simulink model "Batman_Code"  (Simulink 7.8)
settings: Solver=FixedStepDiscrete  StartTime=0.0  StopTime=3  FixedStep=0.000250  RelTol=1e-3
InitFcn:
  | if (rtwenvironmentmode(bdroot(gcbh)) || ...
  |       exist('sldvisactive','file')~=0 && ...
  |       sldvisactive(bdroot(gcbh)) )
  |    ; %Simulation
  | else
  |   SendTargetStop(); %RTW-Build
  | end
values from neighbouring files (symbols this model uses):
  A = diag([ 1  (1-T_s/(C_dl*R_dl))])    [Batman_Code_param.m]
  A_T = A'    [Batman_Code_param.m]
  B = [(T_s/C_cell);  (T_s/C_dl) ]    [Batman_Code_param.m]
  CellNo = uint8(12)    [Batman_Code_param.m]    (also in Init_file_Bat.m = uint16(12))
  I_max_line = int32(100000)    [Batman_Code_param.m]    (also in Init_file_Bat.m = int32(10000))
  I_min_line = int32(-100000)    [Batman_Code_param.m]    (also in Init_file_Bat.m = int32(-10000))
  max_delta_V_cell = uint16(100)    [Batman_Code_param.m]
  p = [2.2966e-006 -3.6644e-004 0.0252 2.9036]'    [Batman_Code_param.m]
  P_0 = [1e-5 8e-8; 8e-8 1.4e-8]    [Batman_Code_param.m]
  Q = diag( B.^2 .* stddev_I_k^2 )    [Batman_Code_param.m]
  R = stddev_V_k^2    (= 1.00195407867e-06)    [Batman_Code_param.m]
  R_i = 0.05    [Batman_Code_param.m]    (also in Init_file_Bat.m = 0.002)
  T_max_cell = uint16(373)    [Batman_Code_param.m]    (also in Init_file_Bat.m)
  T_min_cell = uint16(273)    [Batman_Code_param.m]    (also in Init_file_Bat.m)
  V_max_bat = uint16(49200)    [Batman_Code_param.m]    (also in Init_file_Bat.m = uint16(49080))
  V_max_cell = uint16(4090)    [Batman_Code_param.m]    (also in Init_file_Bat.m)
  V_min_bat = uint16(30000)    [Batman_Code_param.m]    (also in Init_file_Bat.m = uint16(36000))
  V_min_cell = uint16(3000)    [Batman_Code_param.m]    (also in Init_file_Bat.m = uint16(2800))
undefined symbols (not defined in the file or in its folder): BlockLoadFcnInfoBlock
libraries: c280xlib x20, lucasnuelle x2, idelinklib_ticcs x1, c2833xlib x1, idelinklib_tgtpref x1, idelinklib_common x1
(part 1 of 2)
settings Model: Creator=mathlab  LastModifiedBy=user  BufferReuse=off
settings SolverCC: AutoInsertRateTranBlk=on
settings DataIOCC: SaveOutput=off  SaveTime=off
settings OptimizationCC: BlockReduction=off  InlineParams=on  BufferReuse=off  OptimizeModelRefInitCode=on  LifeSpan=1
settings DebuggingCC: MultiTaskDSMMsg=none  MultiTaskCondExecSysMsg=none  UniqueDataStoreMsg=warning  SFNoUnconditionalDefaultTransitionDiag=none
settings HardwareCC: ProdBitPerChar=16  ProdBitPerInt=16  ProdBitPerPointer=16  ProdLargestAtomicInteger=Integer  ProdIntDivRoundTo=Zero  ProdEndianess=LittleEndian  ProdWordSize=16  ProdHWDeviceType=Texas Instruments->C2000
settings RTWCC: SystemTargetFile=idelink_ert.tlc  TLCOptions=-v  GenerateMakefile=off  TemplateMakefile=idelink_ert.tmf  PostCodeGenCommand=LNPostCodeGenCommand(modelName, buildInfo)  Description=IDE Link ERT  ProcessScript=idelink_ert_make_rtw_hook
settings CodeAppCC: IgnoreCustomStorageClasses=off
settings ERTFactory: TargetFcnLib=ansi_tfl_table_tmw.mat  TargetFunctionLibrary=ANSI_C  UtilityFuncGeneration=Auto  ERTMultiwordTypeDef=System defined  CodeExecutionProfiling=off  ERTMultiwordLength=256  MultiwordLength=2048  GenerateFullHeader=on  GenerateSampleERTMain=off  GenerateTestInterfaces=off  IsPILTarget=off  ModelReferenceCompliant=on  ParMdlRefBuildCompliant=off  CompOptLevelCompliant=off  ConcurrentExecutionCompliant=on  IncludeMdlTerminateFcn=on  GeneratePreprocessorConditionals=Disable all  CombineOutputUpdateFcns=on  CombineSignalStateStructs=off  SuppressErrorStatus=off  ERTFirstTimeCompliant=on  IncludeFileDelimiter=Auto  ERTCustomFileBanners=on  SupportAbsoluteTime=on  LogVarNameModifier=rt_  MatFileLogging=off  MultiInstanceERTCode=off  SupportNonFinite=on  SupportComplex=on  PurelyIntegerCode=off  SupportContinuousTime=off  SupportNonInlinedSFcns=on  SupportVariableSizeSignals=off  EnableShiftOperators=on  ParenthesesLevel=Nominal  PortableWordSizes=off  ModelStepFunctionPrototypeControlCompliant=on  CPPClassGenCompliant=off  AutosarCompliant=off  GenerateErtSFunction=off  CreateSILPILBlock=None  CodeExecutionProfileVariable=executionProfile  CodeProfilingSaveOptions=SummaryOnly  GenerateASAP2=off  ExtMode=off  ExtModeTransport=0  ExtModeStaticAlloc=off  ExtModeStaticAllocSize=1000000  ExtModeTesting=off  ExtModeMexFile=TIC2000ExternalModeOpen  ExtModeIntrfLevel=Level2 - Open  InlinedParameterPlacement=Hierarchical  TargetOS=BareBoardExample  MultiInstanceErrorCode=Error  RateGroupingCode=on  RootIOFormat=Individual arguments  RTWCAPISignals=off  RTWCAPIParams=off  RTWCAPIStates=off  RTWCAPIRootIO=off  ERTSrcFileBannerTemplate=ert_code_template.cgt  ERTHdrFileBannerTemplate=ert_code_template.cgt  ERTDataSrcFileTemplate=ert_code_template.cgt  ERTDataHdrFileTemplate=ert_code_template.cgt  ERTCustomFileTemplate=example_file_process.tlc  CoverageDialogOpen=off  EnableDataOwnership=off  SignalDisplayLevel=10  ParamTuneLevel=10  GlobalDataDefinition=Auto  DataDefinitionFile=global.c  GlobalDataReference=Auto  ERTFilePackagingFormat=Modular  DataReferenceFile=global.h  GRTInterface=off  PreserveExpressionOrder=off  PreserveIfCondition=off  ConvertIfToSwitch=off  PreserveExternInFcnDecls=on  SuppressUnreachableDefaultCases=off  EnableUserReplacementTypes=off  MemSecPackage=--- None ---  MemSecDataConstants=Default  MemSecDataIO=Default  MemSecDataInternal=Default  MemSecDataParameters=Default  MemSecFuncInitTerm=Default  MemSecFuncExecute=Default  MemSecFuncSharedUtil=Default  CodeProfilingInstrumentation=off  AdaptorName=Texas Instruments Code Composer Studio v4 (makefile generation only)  exportIDEObj=on  ideObjName=IDE_Obj  oldideObjName=IDE_Obj  ideObjTimeout=1000  oldideObjTimeout=1000  ideObjBuildTimeout=1000  oldideObjBuildTimeout=1000  ProfileGenCode=off  profileBy=Tasks  ProfileNumSamples=100  InlineDSPBlks=off  projectOptions=Release  debugCompilerOptions=-s -O2 -dDSP=1  releaseCompilerOptions=-s -O2 -dDSP=1  compilerOptionsStr=-s -O2 -dDSP=1  getCompilerOptions=off  resetCompilerOptions=off  debugLinkerOptions=-heap0x10000 -ecode_start -q  releaseLinkerOptions=-heap0x10000 -ecode_start -q  linkerOptionsStr=-heap0x10000 -ecode_start -q  getLinkerOptions=off  resetLinkerOptions=off  systemStackSize=600  systemHeapSize=512  buildFormat=Makefile  buildAction=Create  overrunNotificationMethod=None  overrunNotificationFcn=myfunction  oldoverrunNotificationFcn=myfunction  configurePIL=off  configPILBlockAction=None  DiagnosticActions=warning

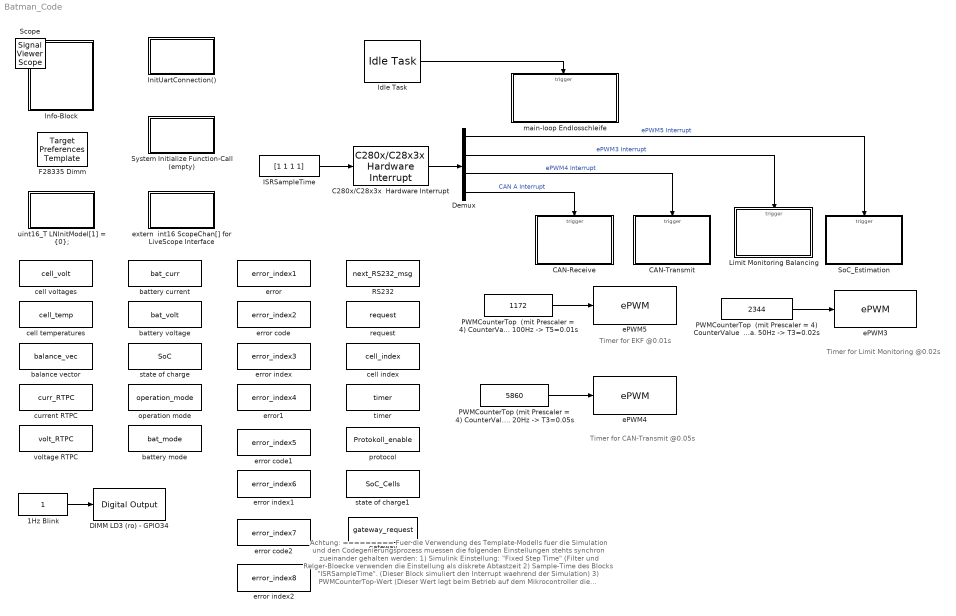
== system Batman_Code ==
  note: Achtung:
      | =========
      | Fuer die Verwendung des Template-Modells fuer die Simulation und den Codegenierungsprozess
      | muessen die folgenden Einstellungen stehts synchron zueinander gehalten werden:
      |
      | 1) Simulink Einstellung: "Fixed Step Time"          (Filter und Relger-Bloecke verwenden die Einstellung als diskrete Abtastzeit
      | 2) Sample-Time des Blocks "ISRSampleTime".   (Dieser Block simuliert den Interrupt waehrend der Simulation)
      | 3) PWMCounterTop-Wert                                    (Dieser Wert legt beim Betrieb auf dem Mikrocontroller die Interrupt-Aufrufzeit fest)
      |                                                                            --> Wert = 150Mhz/(4 * FREQUENZ)
      | Beispiel 4kHz:
      | -------------------------
      | Simulink-Einstellung "FixedStep Time":  0.000250
      | Sample-Time ISRSampleTime-Block:     0.000250
      | PWMCounterTop:                                 150Mhz/(4*4kHz) = 9375
      |
      | Achtung:
      | ==========
      | Werden mehrere Interrupt-Service-Routinen verwendet (hinzugefuegt) muss in jede ISR (Subsystem) der Block: "System Output",
      | wie dieser in den bereits vorhandenen ISRs vorkommt kopiert werden, damit die Oszilloskopfunktion die hoechste Prioritaet besitzt!
  note: Timer for EKF @0.01s
  note: Timer for Limit
      | Monitoring @0.02s
  note: Timer for
      | CAN-Transmit @0.05s
  1Hz Blink : Constant  SampleTime=1
  C280x/C28x3x  Hardware Interrupt : idelinklib_ticcs/C280x//C28x3x Hardware Interrupt  irqnumbers=[3 3 3 9]  pienumbers=[5 3 4 6]  irqpriorities=[99 97 90 80]  irqpreempts=[0 1 0 1]  showinput=on  dspchiptype=C280X
  CAN-Receive : Subsystem  TreatAsAtomicUnit=on
  CAN-Transmit : Subsystem  TreatAsAtomicUnit=on
  DIMM LD3 (ro) - GPIO34 : c2833xlib/Digital Output  GPIO_Number=GPIO32~GPIO39  GPIO_Bit0=off  GPIO_BIT0_Toggle=off  GPIO_Bit1=off  GPIO_BIT1_Toggle=off  GPIO_Bit2=on  GPIO_BIT2_Toggle=on  GPIO_Bit3=off  GPIO_BIT3_Toggle=off  GPIO_Bit4=off  GPIO_BIT4_Toggle=off  GPIO_Bit5=off  GPIO_BIT5_Toggle=off  GPIO_Bit6=off  GPIO_BIT6_Toggle=off  GPIO_Bit7=off  GPIO_BIT7_Toggle=off
  Demux : Demux
  F28335 Dimm : idelinklib_tgtpref/Target Preferences Template  Tag=ccslinktgtpref_ccsv4  library=off
  ISRSampleTime : Constant  Value=[1 1 1 1]  SampleTime=0.000250
  Idle Task : idelinklib_common/Idle Task  tasknumbers=[1]  taskpriorities=100017  taskpreempts=[1]  showinput=off  simPriority=0
  Info-Block : Subsystem  LoadFcn=BlockLoadFcnInfoBlock(gcb);  TreatAsAtomicUnit=on  mask{version=unused, date=unused, modelDescription=unused, hardware=unused, comInterface=LNComFTDI2232, displaySupport=unused, ccssupport=Code Composer Studio 5 (Lucas-Nülle Support), ccstargetconfiguration=C2000 F28335 XDS100V1, ccsmemorymap=F28335 bulk ram}
      mask prompts: version "Modell-Version:"; date "Build-Date:"; modelDescription "Description:"; hardware "Usage for Hardware:"; comInterface "Communication-Interface:"; displaySupport "Display Support:"; ccssupport "Code Composer Studio Support:"; ccstargetconfiguration "Target Configuration:"; ccsmemorymap "Used Memory Map Configuration:"
      mask init:
      | set_param(gcb, 'MaskSelfModifiable', 'on');
      mask StyleString: edit,edit,edit,edit,edit,edit,popup(Code Composer Studio 3.3|Code Composer Studio 5 (Lucas-Nülle Support)),popup(C2000 F28335 XDS100V2|C2000 F28335 XDS100V1|C2000 F28335 XDS100V3|C2000 F28335 XDS200USB|C2000 F28335 XDS510LC|C2000 F28335 XDS510USB|C2000 F28335 XDS560V2USB),popup(System Settings|F28335 External SRAM 512kB|F28335 bulk flash|F28335 bulk ram)
  InitUartConnection() : Subsystem  mask(System Initialize){ShowInLibBrowser=0}
      mask prompts: ShowInLibBrowser "Mask Parameter 1:"
      mask help: Add code to a systems Initialize function
      settings: CopyFcn=cccopyfcn(gcb)  OpenFcn=ccopenfcn('System Initialize Function')
      mask Help: eval('feval(''rtwprivate'',''rtwhelpview'',''rtw_sys_initialize_block'')');
      mask Display: disp('System\nInitialize');
  Limit Monitoring Balancing : Subsystem  TreatAsAtomicUnit=on
  "PWMCounterTop  (mit Prescaler = 4) CounterValue  = 150MHz / (128*10*Freqeuenz) 1172 -> ca. 100Hz -> T5=0.01s" : Constant  Value=1172  OutDataTypeStr=uint32
  "PWMCounterTop  (mit Prescaler = 4) CounterValue  = 150MHz / (128*10*Freqeuenz) 2344 -> ca. 50Hz -> T3=0.02s" : Constant  Value=2344  OutDataTypeStr=uint32
  "PWMCounterTop (mit Prescaler = 4) CounterValue  = 150MHz / (128*10*Freqeuenz) 5860 -> ca. 20Hz -> T3=0.05s" : Constant  Value=5860  OutDataTypeStr=uint32
  RS232 : DataStoreMemory  DataStoreName=next_RS232_msg  ReadBeforeWriteMsg=warning  WriteAfterWriteMsg=warning  WriteAfterReadMsg=warning  InitialValue=1  OutDataTypeStr=boolean
  SoC_Estimation : Subsystem  TreatAsAtomicUnit=on
  System Initialize Function-Call (empty) : Subsystem  mask(System Initialize){ShowInLibBrowser=0}
      mask prompts: ShowInLibBrowser "Mask Parameter 1:"
      mask help: Add code to a systems Initialize function
      settings: CopyFcn=cccopyfcn(gcb)  OpenFcn=ccopenfcn('System Initialize Function')
      mask Help: eval('feval(''rtwprivate'',''rtwhelpview'',''rtw_sys_initialize_block'')');
      mask Display: disp('System\nInitialize');
  balance vector : DataStoreMemory  DataStoreName=balance_vec  ReadBeforeWriteMsg=warning  WriteAfterWriteMsg=warning  WriteAfterReadMsg=warning  InitialValue=zeros(CellNo,1)  OutDataTypeStr=uint8
  battery current : DataStoreMemory  DataStoreName=bat_curr  ReadBeforeWriteMsg=warning  WriteAfterWriteMsg=warning  WriteAfterReadMsg=warning  OutDataTypeStr=int16
  battery mode : DataStoreMemory  DataStoreName=bat_mode  ReadBeforeWriteMsg=warning  WriteAfterWriteMsg=warning  WriteAfterReadMsg=warning  InitialValue=1  OutDataTypeStr=uint16
  battery voltage : DataStoreMemory  DataStoreName=bat_volt  ReadBeforeWriteMsg=warning  WriteAfterWriteMsg=warning  WriteAfterReadMsg=warning  OutDataTypeStr=uint16
  cell index : DataStoreMemory  DataStoreName=cell_index  ReadBeforeWriteMsg=warning  WriteAfterWriteMsg=warning  WriteAfterReadMsg=warning  InitialValue=[0 0]  OutDataTypeStr=uint8
  cell temperatures : DataStoreMemory  DataStoreName=cell_temp  ReadBeforeWriteMsg=warning  WriteAfterWriteMsg=warning  WriteAfterReadMsg=warning  InitialValue=zeros(CellNo,1)  OutDataTypeStr=uint16
  "cell voltages " : DataStoreMemory  DataStoreName=cell_volt  ReadBeforeWriteMsg=warning  WriteAfterWriteMsg=warning  WriteAfterReadMsg=warning  InitialValue=zeros(CellNo,1)  OutDataTypeStr=uint16
  current RTPC : DataStoreMemory  DataStoreName=curr_RTPC  ReadBeforeWriteMsg=warning  WriteAfterWriteMsg=warning  WriteAfterReadMsg=warning  InitialValue=500  OutDataTypeStr=int16
  ePWM3 : c280xlib/ePWM  checkMode=off  useModule=ePWM3  periodUnits=Clock cycles  timerSource=Input port  timerPeriod_clk=0  timerPeriod_sec=PwmTsample  countingMode=Up  synchronizationOption=Disable  synchronizationEnable=off  phaseActiveEnable=Disable  phaseDirection=Count down after sync  phaseActive=0  clockPrescale=128  HSclockPrescale=10  ePWMxAStatus=off  CMPAUnits=Percentages  CMPASource=Specify via dialog  CMPAValue_per=50  CMPAValue_clk=5000  ePWMxAactionLogic1=Clear  ePWMxAactionLogic2=Do nothing  ePWMxAactionLogic3=Set  ePWMxAactionLogic4=Do nothing  ePWMxAactionLogic5=Do nothing  ePWMxAactionLogic6=Do nothing  ePWMxALoadMode=Load on CTR=Zero  ePWMxACSFenable=off  ePWMxACSFvalue=Forcing Disable  ePWMxASFreload=Zero  enHRPWM=off  HRPWM_LoadMode=CTR=ZERO  HRPWM_CTLMode=Phase control mode  HRPWM_EDGMode=Both edge  enSFO=on  ePWMxBStatus=off  CMPBUnits=Percentages  CMPBSource=Specify via dialog  CMPBValue_per=0  CMPBValue_clk=0  ePWMxBactionLogic1=Do nothing  ePWMxBactionLogic2=Set  ePWMxBactionLogic3=Do nothing  ePWMxBactionLogic4=Do nothing  ePWMxBactionLogic5=Clear  ePWMxBactionLogic6=Do nothing  ePWMxBLoadMode=Load on CTR=Zero  ePWMxBCSFenable=off  ePWMxBCSFvalue=Forcing Disable  ePWMxBSFreload=Zero  enableDBePWMxA=off  enableDBePWMxB=off  DBpolarity=AH  DBedgeDelay=Positive  DBSource_ePWMxA=ePWMxA  DBSource_ePWMxB=ePWMxA  DBperiodSource=Specify via dialog  REDperiod=0  FEDperiod=0  adcstartModuleA=off  adcrequestEventA=First event  adcstartEventA=CTR=Zero  adcstartModuleB=off  adcrequestEventB=First event  adcstartEventB=CTR=Zero  intEn=on  intPrd=First event  intSel=CTR=PRD  chopperEnable=off  chopperFrequency=1  chopperFirstwidth=1  chopperDuty=12.5%  tripZonesource=Specify via dialog  tzselOSHT1=off  tzselOSHT2=off  tzselOSHT3=off  tzselOSHT4=off  tzselOSHT5=off  tzselOSHT6=off  tzselCBC1=off  tzselCBC2=off  tzselCBC3=off  tzselCBC4=off  tzselCBC5=off  tzselCBC6=off  enTzOstIntr=off  enTzCbcIntr=off  ePWMxAforced=No action  ePWMxBforced=No action  timerPeriod=-1  ePWMxAValue=1  ePWMxBValue=0  tripZoneoption=OSHT
  ePWM4 : c280xlib/ePWM  checkMode=off  useModule=ePWM4  periodUnits=Clock cycles  timerSource=Input port  timerPeriod_clk=0  timerPeriod_sec=PwmTsample  countingMode=Up  synchronizationOption=Disable  synchronizationEnable=off  phaseActiveEnable=Disable  phaseDirection=Count down after sync  phaseActive=0  clockPrescale=128  HSclockPrescale=10  ePWMxAStatus=off  CMPAUnits=Percentages  CMPASource=Specify via dialog  CMPAValue_per=50  CMPAValue_clk=5000  ePWMxAactionLogic1=Clear  ePWMxAactionLogic2=Do nothing  ePWMxAactionLogic3=Set  ePWMxAactionLogic4=Do nothing  ePWMxAactionLogic5=Do nothing  ePWMxAactionLogic6=Do nothing  ePWMxALoadMode=Load on CTR=Zero  ePWMxACSFenable=off  ePWMxACSFvalue=Forcing Disable  ePWMxASFreload=Zero  enHRPWM=off  HRPWM_LoadMode=CTR=ZERO  HRPWM_CTLMode=Phase control mode  HRPWM_EDGMode=Both edge  enSFO=on  ePWMxBStatus=off  CMPBUnits=Percentages  CMPBSource=Specify via dialog  CMPBValue_per=0  CMPBValue_clk=0  ePWMxBactionLogic1=Do nothing  ePWMxBactionLogic2=Set  ePWMxBactionLogic3=Do nothing  ePWMxBactionLogic4=Do nothing  ePWMxBactionLogic5=Clear  ePWMxBactionLogic6=Do nothing  ePWMxBLoadMode=Load on CTR=Zero  ePWMxBCSFenable=off  ePWMxBCSFvalue=Forcing Disable  ePWMxBSFreload=Zero  enableDBePWMxA=off  enableDBePWMxB=off  DBpolarity=AH  DBedgeDelay=Positive  DBSource_ePWMxA=ePWMxA  DBSource_ePWMxB=ePWMxA  DBperiodSource=Specify via dialog  REDperiod=0  FEDperiod=0  adcstartModuleA=off  adcrequestEventA=First event  adcstartEventA=CTR=Zero  adcstartModuleB=off  adcrequestEventB=First event  adcstartEventB=CTR=Zero  intEn=on  intPrd=First event  intSel=CTR=PRD  chopperEnable=off  chopperFrequency=1  chopperFirstwidth=1  chopperDuty=12.5%  tripZonesource=Specify via dialog  tzselOSHT1=off  tzselOSHT2=off  tzselOSHT3=off  tzselOSHT4=off  tzselOSHT5=off  tzselOSHT6=off  tzselCBC1=off  tzselCBC2=off  tzselCBC3=off  tzselCBC4=off  tzselCBC5=off  tzselCBC6=off  enTzOstIntr=off  enTzCbcIntr=off  ePWMxAforced=No action  ePWMxBforced=No action  timerPeriod=-1  ePWMxAValue=1  ePWMxBValue=0  tripZoneoption=OSHT
  ePWM5 : c280xlib/ePWM  checkMode=off  useModule=ePWM5  periodUnits=Clock cycles  timerSource=Input port  timerPeriod_clk=0  timerPeriod_sec=PwmTsample  countingMode=Up  synchronizationOption=Disable  synchronizationEnable=off  phaseActiveEnable=Disable  phaseDirection=Count down after sync  phaseActive=0  clockPrescale=128  HSclockPrescale=10  ePWMxAStatus=off  CMPAUnits=Percentages  CMPASource=Specify via dialog  CMPAValue_per=50  CMPAValue_clk=5000  ePWMxAactionLogic1=Clear  ePWMxAactionLogic2=Do nothing  ePWMxAactionLogic3=Set  ePWMxAactionLogic4=Do nothing  ePWMxAactionLogic5=Do nothing  ePWMxAactionLogic6=Do nothing  ePWMxALoadMode=Load on CTR=Zero  ePWMxACSFenable=off  ePWMxACSFvalue=Forcing Disable  ePWMxASFreload=Zero  enHRPWM=off  HRPWM_LoadMode=CTR=ZERO  HRPWM_CTLMode=Phase control mode  HRPWM_EDGMode=Both edge  enSFO=on  ePWMxBStatus=off  CMPBUnits=Percentages  CMPBSource=Specify via dialog  CMPBValue_per=0  CMPBValue_clk=0  ePWMxBactionLogic1=Do nothing  ePWMxBactionLogic2=Set  ePWMxBactionLogic3=Do nothing  ePWMxBactionLogic4=Do nothing  ePWMxBactionLogic5=Clear  ePWMxBactionLogic6=Do nothing  ePWMxBLoadMode=Load on CTR=Zero  ePWMxBCSFenable=off  ePWMxBCSFvalue=Forcing Disable  ePWMxBSFreload=Zero  enableDBePWMxA=off  enableDBePWMxB=off  DBpolarity=AH  DBedgeDelay=Positive  DBSource_ePWMxA=ePWMxA  DBSource_ePWMxB=ePWMxA  DBperiodSource=Specify via dialog  REDperiod=0  FEDperiod=0  adcstartModuleA=off  adcrequestEventA=First event  adcstartEventA=CTR=Zero  adcstartModuleB=off  adcrequestEventB=First event  adcstartEventB=CTR=Zero  intEn=on  intPrd=First event  intSel=CTR=PRD  chopperEnable=off  chopperFrequency=1  chopperFirstwidth=1  chopperDuty=12.5%  tripZonesource=Specify via dialog  tzselOSHT1=off  tzselOSHT2=off  tzselOSHT3=off  tzselOSHT4=off  tzselOSHT5=off  tzselOSHT6=off  tzselCBC1=off  tzselCBC2=off  tzselCBC3=off  tzselCBC4=off  tzselCBC5=off  tzselCBC6=off  enTzOstIntr=off  enTzCbcIntr=off  ePWMxAforced=No action  ePWMxBforced=No action  timerPeriod=-1  ePWMxAValue=1  ePWMxBValue=0  tripZoneoption=OSHT
  error : DataStoreMemory  DataStoreName=error_index1  ReadBeforeWriteMsg=warning  WriteAfterWriteMsg=warning  WriteAfterReadMsg=warning  OutDataTypeStr=uint16
  error code : DataStoreMemory  DataStoreName=error_index2  ReadBeforeWriteMsg=warning  WriteAfterWriteMsg=warning  WriteAfterReadMsg=warning  OutDataTypeStr=uint16
  error code1 : DataStoreMemory  DataStoreName=error_index5  ReadBeforeWriteMsg=warning  WriteAfterWriteMsg=warning  WriteAfterReadMsg=warning  OutDataTypeStr=uint16
  error code2 : DataStoreMemory  DataStoreName=error_index7  ReadBeforeWriteMsg=warning  WriteAfterWriteMsg=warning  WriteAfterReadMsg=warning  OutDataTypeStr=uint16
  error index : DataStoreMemory  DataStoreName=error_index3  ReadBeforeWriteMsg=warning  WriteAfterWriteMsg=warning  WriteAfterReadMsg=warning  OutDataTypeStr=uint16
  error index1 : DataStoreMemory  DataStoreName=error_index6  ReadBeforeWriteMsg=warning  WriteAfterWriteMsg=warning  WriteAfterReadMsg=warning  OutDataTypeStr=uint16
  error index2 : DataStoreMemory  DataStoreName=error_index8  ReadBeforeWriteMsg=warning  WriteAfterWriteMsg=warning  WriteAfterReadMsg=warning  OutDataTypeStr=uint16
  error1 : DataStoreMemory  DataStoreName=error_index4  ReadBeforeWriteMsg=warning  WriteAfterWriteMsg=warning  WriteAfterReadMsg=warning  OutDataTypeStr=uint16
  extern  int16 ScopeChan[] for LiveScope Interface : Subsystem  mask(Model Header){ShowInLibBrowser=0}
      mask prompts: ShowInLibBrowser "Mask Parameter 1:"
      mask help: Add code to the model .h file
      settings: CopyFcn=cccopyfcn(gcb)  OpenFcn=ccopenfcn('Model Header')
      mask Help: eval('feval(''rtwprivate'',''rtwhelpview'',''rtw_model_header_block'')');
      mask Display: disp('Model\nHeader');
  "gateway " : DataStoreMemory  DataStoreName=gateway_request  ReadBeforeWriteMsg=warning  WriteAfterWriteMsg=warning  WriteAfterReadMsg=warning  OutDataTypeStr=boolean
  main-loop Endlosschleife : Subsystem  TreatAsAtomicUnit=on
  operation mode : DataStoreMemory  DataStoreName=operation_mode  ReadBeforeWriteMsg=warning  WriteAfterWriteMsg=warning  WriteAfterReadMsg=warning  InitialValue=1  OutDataTypeStr=uint16
  protocol : DataStoreMemory  DataStoreName=Protokoll_enable  ReadBeforeWriteMsg=warning  WriteAfterWriteMsg=warning  WriteAfterReadMsg=warning  InitialValue=zeros(8,1)  OutDataTypeStr=boolean
  request : DataStoreMemory  DataStoreName=request  ReadBeforeWriteMsg=warning  WriteAfterWriteMsg=warning  WriteAfterReadMsg=warning  OutDataTypeStr=uint8
  state of charge : DataStoreMemory  DataStoreName=SoC  ReadBeforeWriteMsg=warning  WriteAfterWriteMsg=warning  WriteAfterReadMsg=warning  OutDataTypeStr=uint16
  state of charge1 : DataStoreMemory  DataStoreName=SoC_Cells  ReadBeforeWriteMsg=warning  WriteAfterWriteMsg=warning  WriteAfterReadMsg=warning  InitialValue=zeros(CellNo,1)  OutDataTypeStr=uint16
  timer : DataStoreMemory  DataStoreName=timer  ReadBeforeWriteMsg=warning  WriteAfterWriteMsg=warning  WriteAfterReadMsg=warning  OutDataTypeStr=uint32
  "uint16_T LNInitModel[1] = {0};" : Subsystem  mask(Model Source){ShowInLibBrowser=0}
      mask prompts: ShowInLibBrowser "Mask Parameter 1:"
      mask help: Add code to the model .c file
      settings: CopyFcn=cccopyfcn(gcb)  OpenFcn=ccopenfcn('Model Source')
      mask Help: eval('feval(''rtwprivate'',''rtwhelpview'',''rtw_model_source_block'')');
      mask Display: disp('Model\nSource');
  voltage RTPC : DataStoreMemory  DataStoreName=volt_RTPC  ReadBeforeWriteMsg=warning  WriteAfterWriteMsg=warning  WriteAfterReadMsg=warning  InitialValue=38000  OutDataTypeStr=uint16
  Scope : SignalViewerScope  IOType=viewer  RefreshTime=0.035000
  wires:
  Idle Task/1 -> main-loop Endlosschleife/Trigger
  "PWMCounterTop  (mit Prescaler = 4) CounterValue  = 150MHz / (128*10*Freqeuenz) 1172 -> ca. 100Hz -> T5=0.01s"/1 -> ePWM5/1
  ISRSampleTime/1 -> C280x/C28x3x  Hardware Interrupt/1
  1Hz Blink/1 -> DIMM LD3 (ro) - GPIO34/1
  "PWMCounterTop  (mit Prescaler = 4) CounterValue  = 150MHz / (128*10*Freqeuenz) 2344 -> ca. 50Hz -> T3=0.02s"/1 -> ePWM3/1
  "PWMCounterTop (mit Prescaler = 4) CounterValue  = 150MHz / (128*10*Freqeuenz) 5860 -> ca. 20Hz -> T3=0.05s"/1 -> ePWM4/1
  C280x/C28x3x  Hardware Interrupt/1 -> Demux/1
  Demux/1 -> SoC_Estimation/Trigger  "ePWM5 Interrupt"
  Demux/2 -> Limit Monitoring Balancing/Trigger  "ePWM3 Interrupt"
  Demux/3 -> CAN-Transmit/Trigger  "ePWM4 Interrupt"
  Demux/4 -> CAN-Receive/Trigger  "CAN A Interrupt"

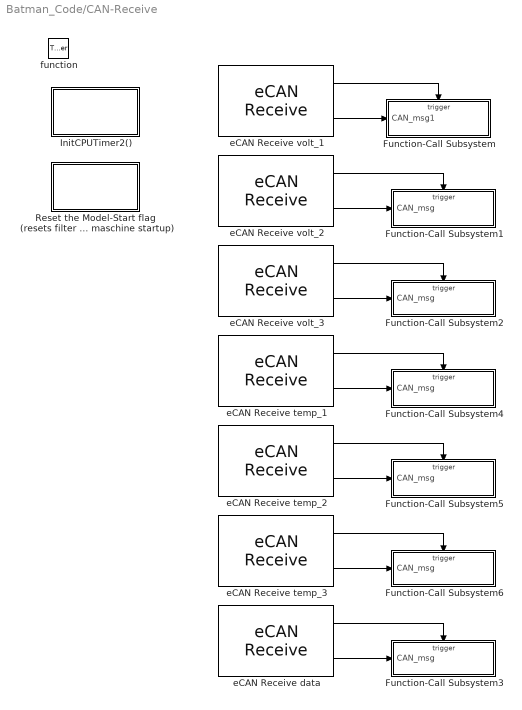
== system Batman_Code/CAN-Receive ==
  function : TriggerPort  TriggerType=function-call  SampleTime=-1
  Function-Call Subsystem : Subsystem  TreatAsAtomicUnit=on
  Function-Call Subsystem1 : Subsystem  TreatAsAtomicUnit=on
  Function-Call Subsystem2 : Subsystem  TreatAsAtomicUnit=on
  Function-Call Subsystem3 : Subsystem  TreatAsAtomicUnit=on
  Function-Call Subsystem4 : Subsystem  TreatAsAtomicUnit=on
  Function-Call Subsystem5 : Subsystem  TreatAsAtomicUnit=on
  Function-Call Subsystem6 : Subsystem  TreatAsAtomicUnit=on
  InitCPUTimer2() : Subsystem  mask(System Outputs){ShowInLibBrowser=0}
      mask prompts: ShowInLibBrowser "Mask Parameter 1:"
      mask help: Add code to a systems Outputs function
      settings: CopyFcn=cccopyfcn(gcb)  OpenFcn=ccopenfcn('System Outputs Function')
      mask Help: eval('feval(''rtwprivate'',''rtwhelpview'',''rtw_sys_outputs_block'')');
      mask Display: disp('System\nOutputs');
  Reset the Model-Start flag  (resets filter and  internal states on state  maschine startup) : Subsystem  mask(System Update){ShowInLibBrowser=0}
      mask prompts: ShowInLibBrowser "Mask Parameter 1:"
      mask help: Add code to a systems Update function
      settings: CopyFcn=cccopyfcn(gcb)  OpenFcn=ccopenfcn('System Update Function')
      mask Help: eval('feval(''rtwprivate'',''rtwhelpview'',''rtw_sys_update_block'')');
      mask Display: disp('System\nUpdate');
  eCAN Receive data : c280xlib/eCAN Receive  chipFamily=C28x3x  useModule=eCAN_A  mailboxNo=7  messageID=id_data_receive_data  messageType=Standard (11-bit identifier)  sampleTime=-1  dataType=uint32  initValue=0  outputMessageLength=off  outputMessageTimeStamp=off  postInterrupt=on  interruptLine=1
  eCAN Receive temp_1 : c280xlib/eCAN Receive  chipFamily=C28x3x  useModule=eCAN_A  mailboxNo=4  messageID=id_data_receive_temperature_1  messageType=Standard (11-bit identifier)  sampleTime=-1  dataType=uint32  initValue=0  outputMessageLength=off  outputMessageTimeStamp=off  postInterrupt=on  interruptLine=1
  eCAN Receive temp_2 : c280xlib/eCAN Receive  chipFamily=C28x3x  useModule=eCAN_A  mailboxNo=5  messageID=id_data_receive_temperature_2  messageType=Standard (11-bit identifier)  sampleTime=-1  dataType=uint32  initValue=0  outputMessageLength=off  outputMessageTimeStamp=off  postInterrupt=on  interruptLine=1
  eCAN Receive temp_3 : c280xlib/eCAN Receive  chipFamily=C28x3x  useModule=eCAN_A  mailboxNo=6  messageID=id_data_receive_temperature_3  messageType=Standard (11-bit identifier)  sampleTime=-1  dataType=uint32  initValue=0  outputMessageLength=off  outputMessageTimeStamp=off  postInterrupt=on  interruptLine=1
  eCAN Receive volt_1 : c280xlib/eCAN Receive  chipFamily=C28x3x  useModule=eCAN_A  mailboxNo=1  messageID=id_data_receive_voltage_1  messageType=Standard (11-bit identifier)  sampleTime=-1  dataType=uint32  initValue=0  outputMessageLength=off  outputMessageTimeStamp=off  postInterrupt=on  interruptLine=1
  eCAN Receive volt_2 : c280xlib/eCAN Receive  chipFamily=C28x3x  useModule=eCAN_A  mailboxNo=2  messageID=id_data_receive_voltage_2  messageType=Standard (11-bit identifier)  sampleTime=-1  dataType=uint32  initValue=0  outputMessageLength=off  outputMessageTimeStamp=off  postInterrupt=on  interruptLine=1
  eCAN Receive volt_3 : c280xlib/eCAN Receive  chipFamily=C28x3x  useModule=eCAN_A  mailboxNo=3  messageID=id_data_receive_voltage_3  messageType=Standard (11-bit identifier)  sampleTime=-1  dataType=uint32  initValue=0  outputMessageLength=off  outputMessageTimeStamp=off  postInterrupt=on  interruptLine=1
  wires:
  eCAN Receive volt_1/1 -> Function-Call Subsystem/Trigger
  eCAN Receive volt_1/2 -> Function-Call Subsystem/1(CAN_msg1)
  eCAN Receive volt_2/1 -> Function-Call Subsystem1/Trigger
  eCAN Receive volt_2/2 -> Function-Call Subsystem1/1(CAN_msg)
  eCAN Receive volt_3/1 -> Function-Call Subsystem2/Trigger
  eCAN Receive volt_3/2 -> Function-Call Subsystem2/1(CAN_msg)
  eCAN Receive data/1 -> Function-Call Subsystem3/Trigger
  eCAN Receive data/2 -> Function-Call Subsystem3/1(CAN_msg)
  eCAN Receive temp_1/1 -> Function-Call Subsystem4/Trigger
  eCAN Receive temp_1/2 -> Function-Call Subsystem4/1(CAN_msg)
  eCAN Receive temp_2/1 -> Function-Call Subsystem5/Trigger
  eCAN Receive temp_2/2 -> Function-Call Subsystem5/1(CAN_msg)
  eCAN Receive temp_3/1 -> Function-Call Subsystem6/Trigger
  eCAN Receive temp_3/2 -> Function-Call Subsystem6/1(CAN_msg)

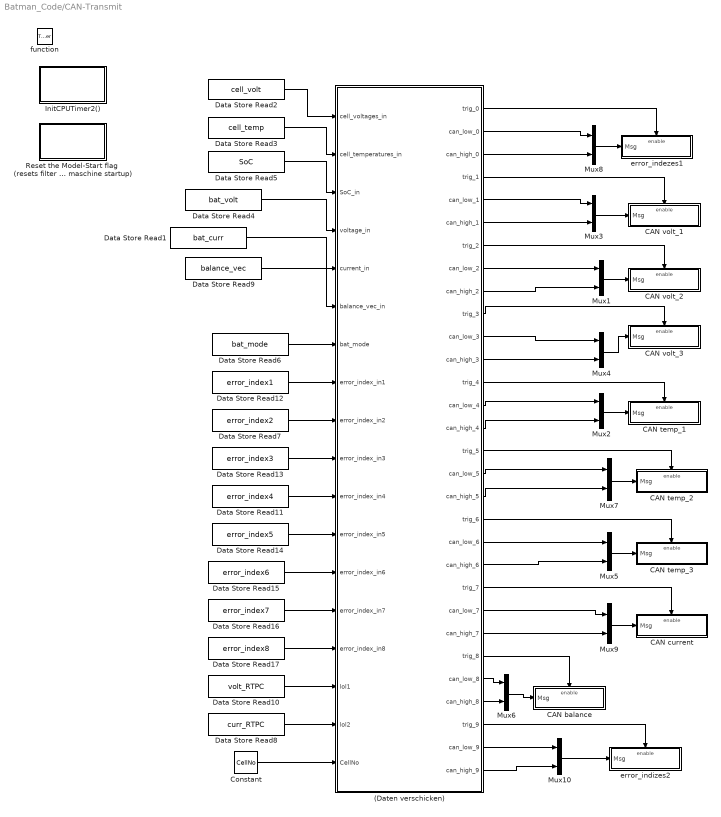
== system Batman_Code/CAN-Transmit ==
  function : TriggerPort  TriggerType=function-call  SampleTime=-1
  (Daten verschicken) : MATLAB Function  TreatAsAtomicUnit=on
  CAN balance : Subsystem  TreatAsAtomicUnit=on
  CAN current : Subsystem  TreatAsAtomicUnit=on
  CAN temp_1 : Subsystem  TreatAsAtomicUnit=on
  CAN temp_2 : Subsystem  TreatAsAtomicUnit=on
  CAN temp_3 : Subsystem  TreatAsAtomicUnit=on
  CAN volt_1 : Subsystem  TreatAsAtomicUnit=on
  CAN volt_2 : Subsystem  TreatAsAtomicUnit=on
  CAN volt_3 : Subsystem  TreatAsAtomicUnit=on
  Constant : Constant  Value=CellNo
  Data Store Read1 : DataStoreRead  DataStoreName=bat_curr
  Data Store Read10 : DataStoreRead  DataStoreName=volt_RTPC
  Data Store Read11 : DataStoreRead  DataStoreName=error_index4
  Data Store Read12 : DataStoreRead  DataStoreName=error_index1
  Data Store Read13 : DataStoreRead  DataStoreName=error_index3
  Data Store Read14 : DataStoreRead  DataStoreName=error_index5
  Data Store Read15 : DataStoreRead  DataStoreName=error_index6
  Data Store Read16 : DataStoreRead  DataStoreName=error_index7
  Data Store Read17 : DataStoreRead  DataStoreName=error_index8
  Data Store Read2 : DataStoreRead  DataStoreName=cell_volt
  Data Store Read3 : DataStoreRead  DataStoreName=cell_temp
  Data Store Read4 : DataStoreRead  DataStoreName=bat_volt
  Data Store Read5 : DataStoreRead  DataStoreName=SoC
  Data Store Read6 : DataStoreRead  DataStoreName=bat_mode
  Data Store Read7 : DataStoreRead  DataStoreName=error_index2
  Data Store Read8 : DataStoreRead  DataStoreName=curr_RTPC
  Data Store Read9 : DataStoreRead  DataStoreName=balance_vec
  InitCPUTimer2() : Subsystem  mask(System Outputs){ShowInLibBrowser=0}
      mask prompts: ShowInLibBrowser "Mask Parameter 1:"
      mask help: Add code to a systems Outputs function
      settings: CopyFcn=cccopyfcn(gcb)  OpenFcn=ccopenfcn('System Outputs Function')
      mask Help: eval('feval(''rtwprivate'',''rtwhelpview'',''rtw_sys_outputs_block'')');
      mask Display: disp('System\nOutputs');
  Mux{1..10} (10 alike) : Mux  Inputs=2
  Reset the Model-Start flag  (resets filter and  internal states on state  maschine startup) : Subsystem  mask(System Update){ShowInLibBrowser=0}
      mask prompts: ShowInLibBrowser "Mask Parameter 1:"
      mask help: Add code to a systems Update function
      settings: CopyFcn=cccopyfcn(gcb)  OpenFcn=ccopenfcn('System Update Function')
      mask Help: eval('feval(''rtwprivate'',''rtwhelpview'',''rtw_sys_update_block'')');
      mask Display: disp('System\nUpdate');
  error_indezes1 : Subsystem  TreatAsAtomicUnit=on
  error_indizes2 : Subsystem  TreatAsAtomicUnit=on
  wires:
  Mux3/1 -> CAN volt_1/1(Msg)
  Mux1/1 -> CAN volt_2/1(Msg)
  Mux4/1 -> CAN volt_3/1(Msg)
  Mux2/1 -> CAN temp_1/1(Msg)
  Mux7/1 -> CAN temp_2/1(Msg)
  Mux5/1 -> CAN temp_3/1(Msg)
  Mux9/1 -> CAN current/1(Msg)
  Mux8/1 -> error_indezes1/1(Msg)
  Mux6/1 -> CAN balance/1(Msg)
  (Daten verschicken)/2(can_low_0) -> Mux8/1
  (Daten verschicken)/3(can_high_0) -> Mux8/2
  (Daten verschicken)/1(trig_0) -> error_indezes1/Enable
  (Daten verschicken)/5(can_low_1) -> Mux3/1
  (Daten verschicken)/6(can_high_1) -> Mux3/2
  (Daten verschicken)/4(trig_1) -> CAN volt_1/Enable
  (Daten verschicken)/9(can_high_2) -> Mux1/2
  (Daten verschicken)/8(can_low_2) -> Mux1/1
  (Daten verschicken)/7(trig_2) -> CAN volt_2/Enable
  (Daten verschicken)/11(can_low_3) -> Mux4/1
  (Daten verschicken)/12(can_high_3) -> Mux4/2
  (Daten verschicken)/10(trig_3) -> CAN volt_3/Enable
  (Daten verschicken)/15(can_high_4) -> Mux2/2
  (Daten verschicken)/14(can_low_4) -> Mux2/1
  (Daten verschicken)/13(trig_4) -> CAN temp_1/Enable
  (Daten verschicken)/17(can_low_5) -> Mux7/1
  (Daten verschicken)/18(can_high_5) -> Mux7/2
  (Daten verschicken)/16(trig_5) -> CAN temp_2/Enable
  (Daten verschicken)/20(can_low_6) -> Mux5/1
  (Daten verschicken)/21(can_high_6) -> Mux5/2
  (Daten verschicken)/19(trig_6) -> CAN temp_3/Enable
  (Daten verschicken)/23(can_low_7) -> Mux9/1
  (Daten verschicken)/24(can_high_7) -> Mux9/2
  (Daten verschicken)/22(trig_7) -> CAN current/Enable
  (Daten verschicken)/26(can_low_8) -> Mux6/1
  (Daten verschicken)/27(can_high_8) -> Mux6/2
  (Daten verschicken)/25(trig_8) -> CAN balance/Enable
  Data Store Read2/1 -> (Daten verschicken)/1(cell_voltages_in)
  Data Store Read3/1 -> (Daten verschicken)/2(cell_temperatures_in)
  Data Store Read5/1 -> (Daten verschicken)/3(SoC_in)
  Data Store Read4/1 -> (Daten verschicken)/4(voltage_in)
  Data Store Read1/1 -> (Daten verschicken)/5(current_in)
  Data Store Read9/1 -> (Daten verschicken)/6(balance_vec_in)
  Data Store Read6/1 -> (Daten verschicken)/7(bat_mode)
  Data Store Read12/1 -> (Daten verschicken)/8(error_index_in1)
  Data Store Read7/1 -> (Daten verschicken)/9(error_index_in2)
  Data Store Read13/1 -> (Daten verschicken)/10(error_index_in3)
  Data Store Read10/1 -> (Daten verschicken)/16(lol1)
  Data Store Read8/1 -> (Daten verschicken)/17(lol2)
  Constant/1 -> (Daten verschicken)/18(CellNo)
  Data Store Read11/1 -> (Daten verschicken)/11(error_index_in4)
  Data Store Read14/1 -> (Daten verschicken)/12(error_index_in5)
  Data Store Read16/1 -> (Daten verschicken)/14(error_index_in7)
  Data Store Read17/1 -> (Daten verschicken)/15(error_index_in8)
  Data Store Read15/1 -> (Daten verschicken)/13(error_index_in6)
  Mux10/1 -> error_indizes2/1(Msg)
  (Daten verschicken)/29(can_low_9) -> Mux10/1
  (Daten verschicken)/30(can_high_9) -> Mux10/2
  (Daten verschicken)/28(trig_9) -> error_indizes2/Enable

== system Batman_Code/Info-Block ==

== system Batman_Code/InitUartConnection() ==

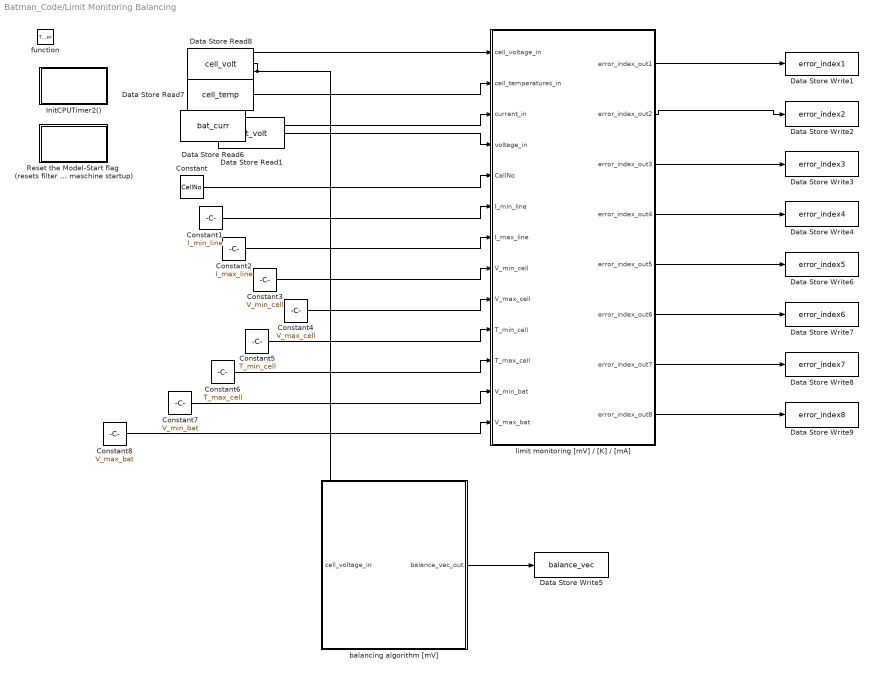
== system Batman_Code/Limit Monitoring Balancing ==
  function : TriggerPort  TriggerType=function-call  SampleTime=-1
  Constant : Constant  Value=CellNo
  Constant1 : Constant  Value=I_min_line
  Constant2 : Constant  Value=I_max_line
  Constant3 : Constant  Value=V_min_cell
  Constant4 : Constant  Value=V_max_cell
  Constant5 : Constant  Value=T_min_cell
  Constant6 : Constant  Value=T_max_cell
  Constant7 : Constant  Value=V_min_bat
  Constant8 : Constant  Value=V_max_bat
  Data Store Read1 : DataStoreRead  DataStoreName=bat_volt
  Data Store Read6 : DataStoreRead  DataStoreName=bat_curr
  Data Store Read7 : DataStoreRead  DataStoreName=cell_temp
  Data Store Read8 : DataStoreRead  DataStoreName=cell_volt
  Data Store Write1 : DataStoreWrite  DataStoreName=error_index1
  Data Store Write2 : DataStoreWrite  DataStoreName=error_index2
  Data Store Write3 : DataStoreWrite  DataStoreName=error_index3
  Data Store Write4 : DataStoreWrite  DataStoreName=error_index4
  Data Store Write5 : DataStoreWrite  DataStoreName=balance_vec
  Data Store Write6 : DataStoreWrite  DataStoreName=error_index5
  Data Store Write7 : DataStoreWrite  DataStoreName=error_index6
  Data Store Write8 : DataStoreWrite  DataStoreName=error_index7
  Data Store Write9 : DataStoreWrite  DataStoreName=error_index8
  InitCPUTimer2() : Subsystem  mask(System Outputs){ShowInLibBrowser=0}
      mask prompts: ShowInLibBrowser "Mask Parameter 1:"
      mask help: Add code to a systems Outputs function
      settings: CopyFcn=cccopyfcn(gcb)  OpenFcn=ccopenfcn('System Outputs Function')
      mask Help: eval('feval(''rtwprivate'',''rtwhelpview'',''rtw_sys_outputs_block'')');
      mask Display: disp('System\nOutputs');
  Reset the Model-Start flag  (resets filter and  internal states on state  maschine startup) : Subsystem  mask(System Update){ShowInLibBrowser=0}
      mask prompts: ShowInLibBrowser "Mask Parameter 1:"
      mask help: Add code to a systems Update function
      settings: CopyFcn=cccopyfcn(gcb)  OpenFcn=ccopenfcn('System Update Function')
      mask Help: eval('feval(''rtwprivate'',''rtwhelpview'',''rtw_sys_update_block'')');
      mask Display: disp('System\nUpdate');
  balancing algorithm [mV] : MATLAB Function  TreatAsAtomicUnit=on
  limit monitoring [mV] / [K] / [mA] : MATLAB Function  TreatAsAtomicUnit=on
  wires:
  Data Store Read6/1 -> limit monitoring [mV] / [K] / [mA]/3(current_in)
  Data Store Read8/1 -> balancing algorithm [mV]/1(cell_voltage_in), limit monitoring [mV] / [K] / [mA]/1(cell_voltage_in)
  Data Store Read7/1 -> limit monitoring [mV] / [K] / [mA]/2(cell_temperatures_in)
  limit monitoring [mV] / [K] / [mA]/1(error_index_out1) -> Data Store Write1/1
  limit monitoring [mV] / [K] / [mA]/2(error_index_out2) -> Data Store Write2/1
  balancing algorithm [mV]/1(balance_vec_out) -> Data Store Write5/1
  limit monitoring [mV] / [K] / [mA]/3(error_index_out3) -> Data Store Write3/1
  Data Store Read1/1 -> limit monitoring [mV] / [K] / [mA]/4(voltage_in)
  Constant1/1 -> limit monitoring [mV] / [K] / [mA]/6(I_min_line)
  Constant/1 -> limit monitoring [mV] / [K] / [mA]/5(CellNo)
  Constant8/1 -> limit monitoring [mV] / [K] / [mA]/13(V_max_bat)
  Constant7/1 -> limit monitoring [mV] / [K] / [mA]/12(V_min_bat)
  Constant6/1 -> limit monitoring [mV] / [K] / [mA]/11(T_max_cell)
  Constant5/1 -> limit monitoring [mV] / [K] / [mA]/10(T_min_cell)
  Constant4/1 -> limit monitoring [mV] / [K] / [mA]/9(V_max_cell)
  Constant3/1 -> limit monitoring [mV] / [K] / [mA]/8(V_min_cell)
  Constant2/1 -> limit monitoring [mV] / [K] / [mA]/7(I_max_line)
  limit monitoring [mV] / [K] / [mA]/4(error_index_out4) -> Data Store Write4/1
  limit monitoring [mV] / [K] / [mA]/5(error_index_out5) -> Data Store Write6/1
  limit monitoring [mV] / [K] / [mA]/7(error_index_out7) -> Data Store Write8/1
  limit monitoring [mV] / [K] / [mA]/8(error_index_out8) -> Data Store Write9/1
  limit monitoring [mV] / [K] / [mA]/6(error_index_out6) -> Data Store Write7/1

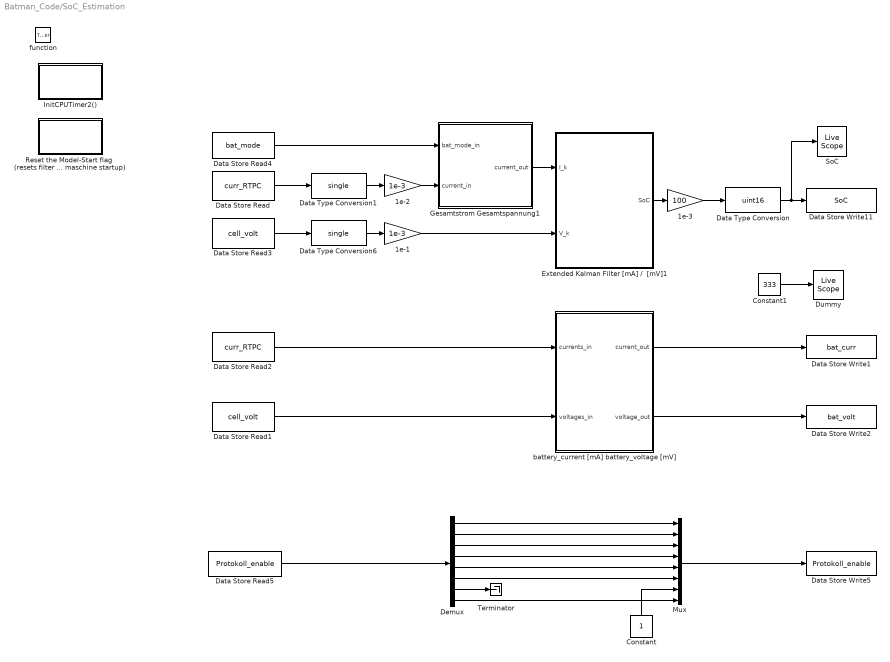
== system Batman_Code/SoC_Estimation ==
  function : TriggerPort  TriggerType=function-call  SampleTime=-1
  1e-1 : Gain  Gain=1e-3
  1e-2 : Gain  Gain=1e-3
  1e-3 : Gain  Gain=100
  Constant : Constant  OutDataTypeStr=boolean
  Constant1 : Constant  Value=333  OutDataTypeStr=uint16
  Data Store Read : DataStoreRead  DataStoreName=curr_RTPC
  Data Store Read1 : DataStoreRead  DataStoreName=cell_volt
  Data Store Read2 : DataStoreRead  DataStoreName=curr_RTPC
  Data Store Read3 : DataStoreRead  DataStoreName=cell_volt
  Data Store Read4 : DataStoreRead  DataStoreName=bat_mode
  Data Store Read5 : DataStoreRead  DataStoreName=Protokoll_enable
  Data Store Write1 : DataStoreWrite  DataStoreName=bat_curr
  Data Store Write11 : DataStoreWrite  DataStoreName=SoC
  Data Store Write2 : DataStoreWrite  DataStoreName=bat_volt
  Data Store Write5 : DataStoreWrite  DataStoreName=Protokoll_enable
  Data Type Conversion : DataTypeConversion  OutDataTypeStr=uint16
  Data Type Conversion1 : DataTypeConversion  OutDataTypeStr=single
  Data Type Conversion6 : DataTypeConversion  OutDataTypeStr=single
  Demux : Demux  Outputs=8
  Dummy : lucasnuelle/Communication/Live Scope  channelNbr=2  DataTypeInput=uint16
  Extended Kalman Filter [mA] /  [mV]1 : MATLAB Function  TreatAsAtomicUnit=on
  Gesamtstrom Gesamtspannung1 : MATLAB Function  TreatAsAtomicUnit=on
  InitCPUTimer2() : Subsystem  mask(System Outputs){ShowInLibBrowser=0}
      mask prompts: ShowInLibBrowser "Mask Parameter 1:"
      mask help: Add code to a systems Outputs function
      settings: CopyFcn=cccopyfcn(gcb)  OpenFcn=ccopenfcn('System Outputs Function')
      mask Help: eval('feval(''rtwprivate'',''rtwhelpview'',''rtw_sys_outputs_block'')');
      mask Display: disp('System\nOutputs');
  Mux : Mux  Inputs=8
  Reset the Model-Start flag  (resets filter and  internal states on state  maschine startup) : Subsystem  mask(System Update){ShowInLibBrowser=0}
      mask prompts: ShowInLibBrowser "Mask Parameter 1:"
      mask help: Add code to a systems Update function
      settings: CopyFcn=cccopyfcn(gcb)  OpenFcn=ccopenfcn('System Update Function')
      mask Help: eval('feval(''rtwprivate'',''rtwhelpview'',''rtw_sys_update_block'')');
      mask Display: disp('System\nUpdate');
  SoC : lucasnuelle/Communication/Live Scope  channelNbr=1  DataTypeInput=uint16
  Terminator : Terminator
  battery_current [mA] battery_voltage [mV] : MATLAB Function  TreatAsAtomicUnit=on
  wires:
  Data Type Conversion/1 -> Data Store Write11/1, SoC/1
  battery_current [mA] battery_voltage [mV]/1(current_out) -> Data Store Write1/1
  Data Type Conversion6/1 -> 1e-1/1
  Data Store Read3/1 -> Data Type Conversion6/1
  Data Store Read2/1 -> battery_current [mA] battery_voltage [mV]/1(currents_in)
  Data Type Conversion1/1 -> 1e-2/1
  Data Store Read4/1 -> Gesamtstrom Gesamtspannung1/1(bat_mode_in)
  1e-2/1 -> Gesamtstrom Gesamtspannung1/2(current_in)
  Gesamtstrom Gesamtspannung1/1(current_out) -> Extended Kalman Filter [mA] /  [mV]1/1(I_k)
  Data Store Read/1 -> Data Type Conversion1/1
  Extended Kalman Filter [mA] /  [mV]1/1(SoC) -> 1e-3/1
  1e-1/1 -> Extended Kalman Filter [mA] /  [mV]1/2(V_k)
  1e-3/1 -> Data Type Conversion/1
  battery_current [mA] battery_voltage [mV]/2(voltage_out) -> Data Store Write2/1
  Data Store Read1/1 -> battery_current [mA] battery_voltage [mV]/2(voltages_in)
  Mux/1 -> Data Store Write5/1
  Data Store Read5/1 -> Demux/1
  Demux/1 -> Mux/1
  Demux/2 -> Mux/2
  Demux/3 -> Mux/3
  Demux/4 -> Mux/4
  Demux/5 -> Mux/5
  Constant/1 -> Mux/7
  Demux/6 -> Mux/6
  Demux/8 -> Mux/8
  Demux/7 -> Terminator/1
  Constant1/1 -> Dummy/1

== system Batman_Code/System Initialize Function-Call (empty) ==

== system Batman_Code/extern  int16 ScopeChan[] for LiveScope Interface ==

== system Batman_Code/main-loop Endlosschleife ==
  function : TriggerPort  TriggerType=function-call
  InitCPUTimer2() : Subsystem  mask(System Outputs){ShowInLibBrowser=0}
      mask prompts: ShowInLibBrowser "Mask Parameter 1:"
      mask help: Add code to a systems Outputs function
      settings: CopyFcn=cccopyfcn(gcb)  OpenFcn=ccopenfcn('System Outputs Function')
      mask Help: eval('feval(''rtwprivate'',''rtwhelpview'',''rtw_sys_outputs_block'')');
      mask Display: disp('System\nOutputs');

== system Batman_Code/uint16_T LNInitModel[1] = {0}; ==

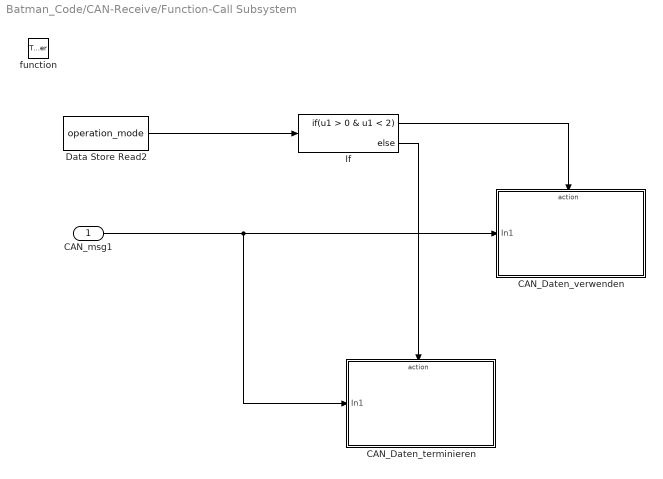
== system Batman_Code/CAN-Receive/Function-Call Subsystem ==
  CAN_msg1 : Inport
  function : TriggerPort  TriggerType=function-call
  CAN_Daten_terminieren : Subsystem  TreatAsAtomicUnit=on
  CAN_Daten_verwenden : Subsystem  TreatAsAtomicUnit=on
  Data Store Read2 : DataStoreRead  DataStoreName=operation_mode
  If : If  IfExpression=u1 > 0 & u1 < 2
  wires:
  If/1 -> CAN_Daten_verwenden/Action
  If/2 -> CAN_Daten_terminieren/Action
  Data Store Read2/1 -> If/1
  CAN_msg1/1 -> CAN_Daten_verwenden/1(In1), CAN_Daten_terminieren/1(In1)

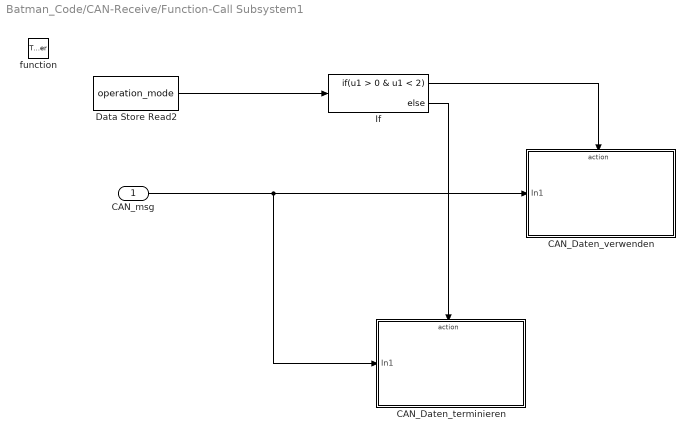
== system Batman_Code/CAN-Receive/Function-Call Subsystem1 ==
  CAN_msg : Inport
  function : TriggerPort  TriggerType=function-call
  CAN_Daten_terminieren : Subsystem  TreatAsAtomicUnit=on
  CAN_Daten_verwenden : Subsystem  TreatAsAtomicUnit=on
  Data Store Read2 : DataStoreRead  DataStoreName=operation_mode
  If : If  IfExpression=u1 > 0 & u1 < 2
  wires:
  If/1 -> CAN_Daten_verwenden/Action
  If/2 -> CAN_Daten_terminieren/Action
  Data Store Read2/1 -> If/1
  CAN_msg/1 -> CAN_Daten_terminieren/1(In1), CAN_Daten_verwenden/1(In1)

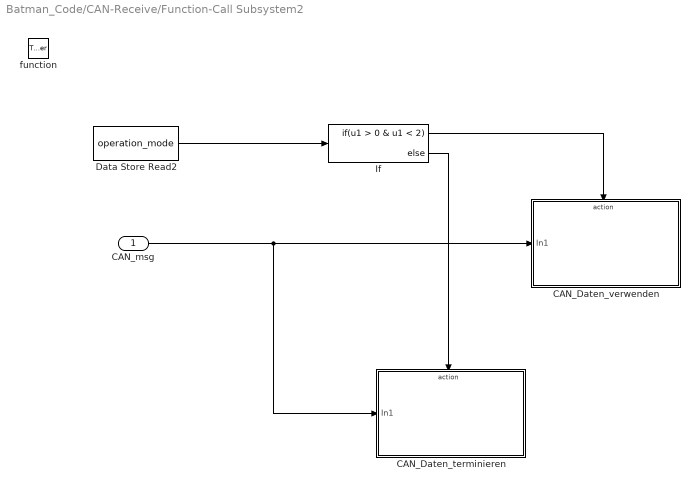
== system Batman_Code/CAN-Receive/Function-Call Subsystem2 ==
  CAN_msg : Inport
  function : TriggerPort  TriggerType=function-call
  CAN_Daten_terminieren : Subsystem  TreatAsAtomicUnit=on
  CAN_Daten_verwenden : Subsystem  TreatAsAtomicUnit=on
  Data Store Read2 : DataStoreRead  DataStoreName=operation_mode
  If : If  IfExpression=u1 > 0 & u1 < 2
  wires:
  If/1 -> CAN_Daten_verwenden/Action
  If/2 -> CAN_Daten_terminieren/Action
  Data Store Read2/1 -> If/1
  CAN_msg/1 -> CAN_Daten_terminieren/1(In1), CAN_Daten_verwenden/1(In1)

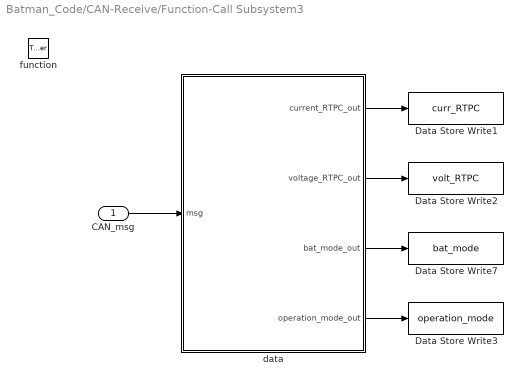
== system Batman_Code/CAN-Receive/Function-Call Subsystem3 ==
  CAN_msg : Inport
  function : TriggerPort  TriggerType=function-call
  Data Store Write1 : DataStoreWrite  DataStoreName=curr_RTPC
  Data Store Write2 : DataStoreWrite  DataStoreName=volt_RTPC
  Data Store Write3 : DataStoreWrite  DataStoreName=operation_mode
  Data Store Write7 : DataStoreWrite  DataStoreName=bat_mode
  data : MATLAB Function  TreatAsAtomicUnit=on
  wires:
  CAN_msg/1 -> data/1(msg)
  data/1(current_RTPC_out) -> Data Store Write1/1
  data/3(bat_mode_out) -> Data Store Write7/1
  data/2(voltage_RTPC_out) -> Data Store Write2/1
  data/4(operation_mode_out) -> Data Store Write3/1

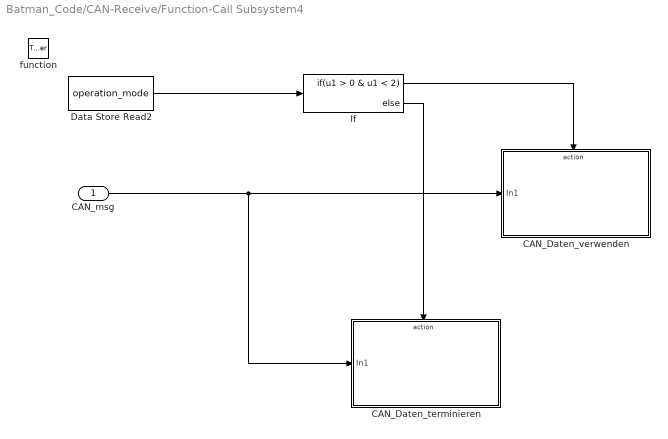
== system Batman_Code/CAN-Receive/Function-Call Subsystem4 ==
  CAN_msg : Inport
  function : TriggerPort  TriggerType=function-call
  CAN_Daten_terminieren : Subsystem  TreatAsAtomicUnit=on
  CAN_Daten_verwenden : Subsystem  TreatAsAtomicUnit=on
  Data Store Read2 : DataStoreRead  DataStoreName=operation_mode
  If : If  IfExpression=u1 > 0 & u1 < 2
  wires:
  If/1 -> CAN_Daten_verwenden/Action
  If/2 -> CAN_Daten_terminieren/Action
  Data Store Read2/1 -> If/1
  CAN_msg/1 -> CAN_Daten_verwenden/1(In1), CAN_Daten_terminieren/1(In1)

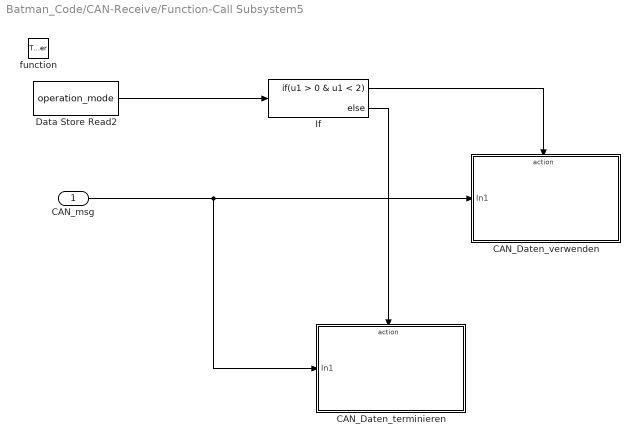
== system Batman_Code/CAN-Receive/Function-Call Subsystem5 ==
  CAN_msg : Inport
  function : TriggerPort  TriggerType=function-call
  CAN_Daten_terminieren : Subsystem  TreatAsAtomicUnit=on
  CAN_Daten_verwenden : Subsystem  TreatAsAtomicUnit=on
  Data Store Read2 : DataStoreRead  DataStoreName=operation_mode
  If : If  IfExpression=u1 > 0 & u1 < 2
  wires:
  If/1 -> CAN_Daten_verwenden/Action
  If/2 -> CAN_Daten_terminieren/Action
  Data Store Read2/1 -> If/1
  CAN_msg/1 -> CAN_Daten_terminieren/1(In1), CAN_Daten_verwenden/1(In1)

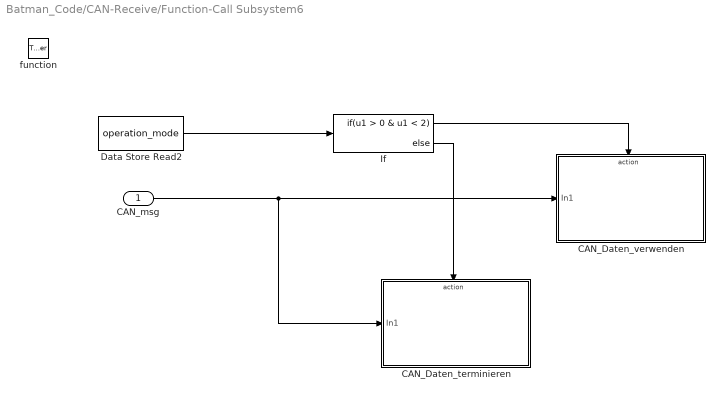
== system Batman_Code/CAN-Receive/Function-Call Subsystem6 ==
  CAN_msg : Inport
  function : TriggerPort  TriggerType=function-call
  CAN_Daten_terminieren : Subsystem  TreatAsAtomicUnit=on
  CAN_Daten_verwenden : Subsystem  TreatAsAtomicUnit=on
  Data Store Read2 : DataStoreRead  DataStoreName=operation_mode
  If : If  IfExpression=u1 > 0 & u1 < 2
  wires:
  If/1 -> CAN_Daten_verwenden/Action
  If/2 -> CAN_Daten_terminieren/Action
  Data Store Read2/1 -> If/1
  CAN_msg/1 -> CAN_Daten_terminieren/1(In1), CAN_Daten_verwenden/1(In1)

== system Batman_Code/CAN-Receive/InitCPUTimer2() ==

== system Batman_Code/CAN-Receive/Reset the Model-Start flag  (resets filter and  internal states on state  maschine startup) ==

== system Batman_Code/CAN-Transmit/CAN balance ==
  Msg : Inport
  Enable : EnablePort
  eCAN Transmit : c280xlib/eCAN Transmit  chipFamily=C280x  useModule=eCAN_A  mailboxNo=18  messageID=id_data_send_balance  messageType=Standard (11-bit identifier)  enableBlockingMode=off  postInterrupt=off  interruptLine=0
  wires:
  Msg/1 -> eCAN Transmit/1

== system Batman_Code/CAN-Transmit/CAN current ==
  Msg : Inport
  Enable : EnablePort
  eCAN Transmit : c280xlib/eCAN Transmit  chipFamily=C28x3x  useModule=eCAN_A  mailboxNo=17  messageID=id_data_send_data  messageType=Standard (11-bit identifier)  enableBlockingMode=off  postInterrupt=off  interruptLine=0
  wires:
  Msg/1 -> eCAN Transmit/1

== system Batman_Code/CAN-Transmit/CAN temp_1 ==
  Msg : Inport
  Enable : EnablePort
  eCAN Transmit : c280xlib/eCAN Transmit  chipFamily=C28x3x  useModule=eCAN_A  mailboxNo=14  messageID=id_data_send_temperature_1  messageType=Standard (11-bit identifier)  enableBlockingMode=off  postInterrupt=off  interruptLine=0
  wires:
  Msg/1 -> eCAN Transmit/1

== system Batman_Code/CAN-Transmit/CAN temp_2 ==
  Msg : Inport
  Enable : EnablePort
  eCAN Transmit : c280xlib/eCAN Transmit  chipFamily=C28x3x  useModule=eCAN_A  mailboxNo=15  messageID=id_data_send_temperature_2  messageType=Standard (11-bit identifier)  enableBlockingMode=off  postInterrupt=off  interruptLine=0
  wires:
  Msg/1 -> eCAN Transmit/1

== system Batman_Code/CAN-Transmit/CAN temp_3 ==
  Msg : Inport
  Enable : EnablePort
  eCAN Transmit : c280xlib/eCAN Transmit  chipFamily=C28x3x  useModule=eCAN_A  mailboxNo=16  messageID=id_data_send_temperature_3  messageType=Standard (11-bit identifier)  enableBlockingMode=off  postInterrupt=off  interruptLine=0
  wires:
  Msg/1 -> eCAN Transmit/1

== system Batman_Code/CAN-Transmit/CAN volt_1 ==
  Msg : Inport
  Enable : EnablePort
  eCAN Transmit : c280xlib/eCAN Transmit  chipFamily=C28x3x  useModule=eCAN_A  mailboxNo=11  messageID=id_data_send_voltage_1  messageType=Standard (11-bit identifier)  enableBlockingMode=off  postInterrupt=off  interruptLine=0
  wires:
  Msg/1 -> eCAN Transmit/1

== system Batman_Code/CAN-Transmit/CAN volt_2 ==
  Msg : Inport
  Enable : EnablePort
  eCAN Transmit : c280xlib/eCAN Transmit  chipFamily=C28x3x  useModule=eCAN_A  mailboxNo=12  messageID=id_data_send_voltage_2  messageType=Standard (11-bit identifier)  enableBlockingMode=off  postInterrupt=off  interruptLine=0
  wires:
  Msg/1 -> eCAN Transmit/1

== system Batman_Code/CAN-Transmit/CAN volt_3 ==
  Msg : Inport
  Enable : EnablePort
  eCAN Transmit : c280xlib/eCAN Transmit  chipFamily=C28x3x  useModule=eCAN_A  mailboxNo=13  messageID=id_data_send_voltage_3  messageType=Standard (11-bit identifier)  enableBlockingMode=off  postInterrupt=off  interruptLine=0
  wires:
  Msg/1 -> eCAN Transmit/1

== system Batman_Code/CAN-Transmit/InitCPUTimer2() ==

== system Batman_Code/CAN-Transmit/Reset the Model-Start flag  (resets filter and  internal states on state  maschine startup) ==

== system Batman_Code/CAN-Transmit/error_indezes1 ==
  Msg : Inport
  Enable : EnablePort
  eCAN Transmit : c280xlib/eCAN Transmit  chipFamily=C28x3x  useModule=eCAN_A  mailboxNo=19  messageID=id_send_error1  messageType=Standard (11-bit identifier)  enableBlockingMode=off  postInterrupt=off  interruptLine=0
  wires:
  Msg/1 -> eCAN Transmit/1

== system Batman_Code/CAN-Transmit/error_indizes2 ==
  Msg : Inport
  Enable : EnablePort
  eCAN Transmit : c280xlib/eCAN Transmit  chipFamily=C280x  useModule=eCAN_A  mailboxNo=20  messageID=id_send_error2  messageType=Standard (11-bit identifier)  enableBlockingMode=off  postInterrupt=off  interruptLine=0
  wires:
  Msg/1 -> eCAN Transmit/1

== system Batman_Code/Limit Monitoring Balancing/InitCPUTimer2() ==
